simulink model "PV_BAT_GRID_TL"  (R2013a)
settings: Solver=ode23t  StartTime=0.0  StopTime=1  RelTol=1e-3
undefined symbols (not defined in the file): Acid, Lead
libraries: powerlib x39, powerlib_meascontrol x10, simulink x4, electricdrivelib x2, fuzblock x2, powerlib_extras x1
settings Model: Creator=penglei  LastModifiedBy=SRIDHARAN
settings SolverCC: ZeroCrossControl=DisableAll
settings DataIOCC: SignalLoggingSaveFormat=ModelDataLogs
settings OptimizationCC: ExpressionDepthLimit=2147483647
settings DebuggingCC: FcnCallInpInsideContextMsg=UseLocalSettings  StrictBusMsg=Warning
settings GRTTargetCC: CombineOutputUpdateFcns=off  GRTInterface=on

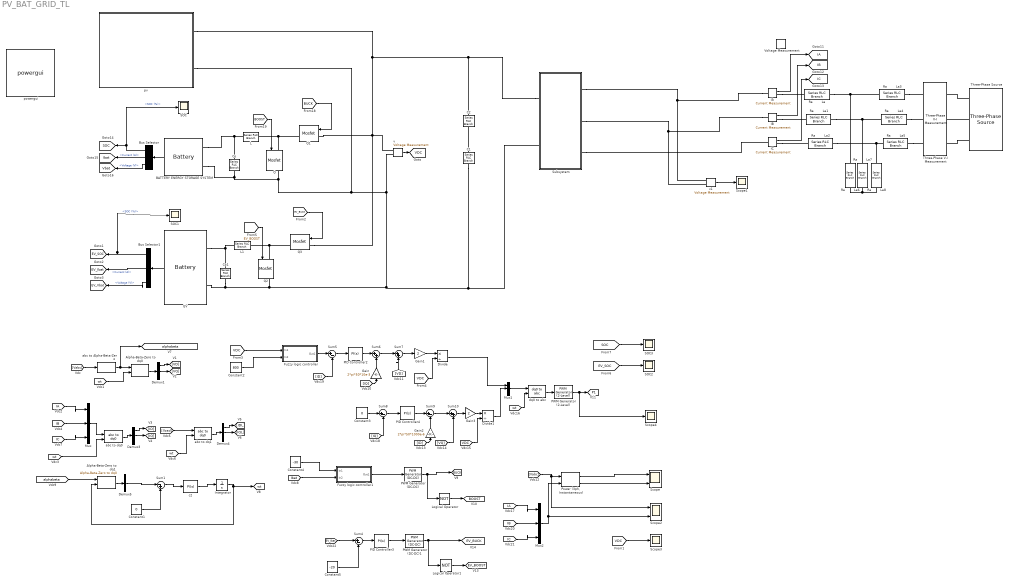
== system PV_BAT_GRID_TL ==
  Alpha-Beta-Zero to dq0 : powerlib_meascontrol/Transformations/Alpha-Beta-Zero to dq0  Alignment=90 degrees behind phase A axis
  Alpha-Beta-Zero to dq1 : powerlib_meascontrol/Transformations/Alpha-Beta-Zero to dq0  Alignment=90 degrees behind phase A axis
  BATTERY ENERGY STORAGE SYSTEM : electricdrivelib/Extra Sources/Battery  BatType=Lead-Acid  ShowDetailedParameters=off  NomV=360  NomQ=300  SOC=50  PresetModel=on  MaxQ=312.5  FullV=391.9737  Dis_rate=60  R=0.012  Normal_OP=93.0833  expZone="[366.5132             1]"  Dis_Char=off  current=[1.5 3]  Units=Ampere-hour  Batt_Tr=1
  Bus Selector : BusSelector  OutputSignals=SOC (%),Current (A),Voltage (V)
  Bus Selector1 : BusSelector  OutputSignals=SOC (%),Current (A),Voltage (V)
  C1 : powerlib/Elements/Series RLC Branch  LConnTagsString=__new0  RConnTagsString=__new0  BranchType=RC  Resistance=1e-3  Inductance=1.0  SetiL0=off  InitialCurrent=0  Capacitance=2500e-6  Setx0=on  InitialVoltage=400  Measurements=None
  C2 : powerlib/Elements/Series RLC Branch  LConnTagsString=__new0  RConnTagsString=__new0  BranchType=RC  Resistance=1e-3  Inductance=1.0  SetiL0=off  InitialCurrent=0  Capacitance=2500e-6  Setx0=on  InitialVoltage=400  Measurements=None
  Co : powerlib/Elements/Series RLC Branch  LConnTagsString=__new0  RConnTagsString=__new0  BranchType=RC  Resistance=0.0001  Inductance=1.0  SetiL0=off  InitialCurrent=0  Capacitance=0.625e-6  Setx0=off  InitialVoltage=0  Measurements=None
  Co1 : powerlib/Elements/Series RLC Branch  LConnTagsString=__new0  RConnTagsString=__new0  BranchType=RC  Resistance=0.0001  Inductance=1.0  SetiL0=off  InitialCurrent=0  Capacitance=0.625e-6  Setx0=off  InitialVoltage=0  Measurements=None
  Constant1 : Constant  Value=0
  Constant2 : Constant  Value=800
  Constant3 : Constant  Value=0
  Constant4 : Constant  Value=-30
  Constant5 : Constant  Value=-20
  Demux{1,3..5} (4 alike) : Demux  Outputs=3
  Divide : Product  Inputs=*/
  Divide1 : Product  Inputs=*/
  EV : electricdrivelib/Extra Sources/Battery  BatType=Lead-Acid  ShowDetailedParameters=off  NomV=48  NomQ=300  SOC=50  PresetModel=on  MaxQ=312.5  FullV=52.2632  Dis_rate=60  R=0.0016  Normal_OP=93.0833  expZone="[48.8684            1]"  Dis_Char=off  current=[1.5 3]  Units=Ampere-hour  Batt_Tr=1
  Fuzzy logic controller : Subsystem
  Fuzzy logic controller1 : Subsystem
  Gain : Gain  Gain=2*pi*50*10e-3
  Gain1 : Gain  Gain=2
  Gain2 : Gain  Gain=2*pi*50*1000e-6
  Gain3 : Gain  Gain=2
  IA : powerlib/Measurements/Current Measurement  PhasorSimulation=off  OutputType=Complex  PSBequivalent=0
  IB : powerlib/Measurements/Current Measurement  PhasorSimulation=off  OutputType=Complex  PSBequivalent=0
  IC : powerlib/Measurements/Current Measurement  PhasorSimulation=off  OutputType=Complex  PSBequivalent=0
  Integrator : Integrator
  L : powerlib/Elements/Series RLC Branch  LConnTagsString=__new0  RConnTagsString=__new0  BranchType=RL  Resistance=0.0001  Inductance=20e-3  SetiL0=off  InitialCurrent=0  Capacitance=1.0  Setx0=off  InitialVoltage=0  Measurements=None
  L1 : powerlib/Elements/Series RLC Branch  LConnTagsString=__new0  RConnTagsString=__new0  BranchType=RL  Resistance=0.0001  Inductance=20e-3  SetiL0=off  InitialCurrent=0  Capacitance=1.0  Setx0=off  InitialVoltage=0  Measurements=None
  Logical Operator : Logic  Operator=NOT  AllPortsSameDT=off  OutDataTypeStr=boolean
  Logical Operator1 : Logic  Operator=NOT  AllPortsSameDT=off  OutDataTypeStr=boolean
  Mux : Mux  Inputs=3
  Mux1 : Mux  Inputs=3
  Mux2 : Mux  Inputs=3
  PID Controller2 : simulink/Continuous/PID Controller  Controller=PI  TimeDomain=Continuous-time  SampleTime=1  IntegratorMethod=Forward Euler  FilterMethod=Forward Euler  Form=Parallel  P=25  I=500  D=0  N=100  InitialConditionSource=internal  InitialConditionForIntegrator=0  InitialConditionForFilter=0  ExternalReset=none  LimitOutput=off  UpperSaturationLimit=1000  LowerSaturationLimit=-1000  LinearizeAsGain=on  AntiWindupMode=none  Kb=1  TrackingMode=off  Kt=1  PParamMin=[]  PParamMax=[]  IParamMin=[]  IParamMax=[]  DParamMin=[]  DParamMax=[]  NParamMin=[]  NParamMax=[]  KbParamMin=[]  KbParamMax=[]  KtParamMin=[]  KtParamMax=[]  POutMin=[]  POutMax=[]  IOutMin=[]  IOutMax=[]  DOutMin=[]  DOutMax=[]  NOutMin=[]  NOutMax=[]  KbOutMin=[]  KbOutMax=[]  KtOutMin=[]  KtOutMax=[]  IntegratorOutMin=[]  IntegratorOutMax=[]  FilterOutMin=[]  FilterOutMax=[]  SumOutMin=[]  SumOutMax=[]  SumI1OutMin=[]  SumI1OutMax=[]  SumI2OutMin=[]  SumI2OutMax=[]  SumI3OutMin=[]  SumI3OutMax=[]  SumDOutMin=[]  SumDOutMax=[]  SaturationOutMin=[]  SaturationOutMax=[]  IntegratorContinuousStateAttributes=''  IntegratorStateMustResolveToSignalObject=off  IntegratorRTWStateStorageClass=Auto  FilterContinuousStateAttributes=''  FilterStateMustResolveToSignalObject=off  FilterRTWStateStorageClass=Auto
  PID Controller3 : simulink/Continuous/PID Controller  Controller=PI  TimeDomain=Continuous-time  SampleTime=1  IntegratorMethod=Forward Euler  FilterMethod=Forward Euler  Form=Parallel  P=0.005  I=10  D=0  N=100  InitialConditionSource=internal  InitialConditionForIntegrator=0  InitialConditionForFilter=0  ExternalReset=none  LimitOutput=on  UpperSaturationLimit=0.95  LowerSaturationLimit=0  LinearizeAsGain=on  AntiWindupMode=none  Kb=1  TrackingMode=off  Kt=1  PParamMin=[]  PParamMax=[]  IParamMin=[]  IParamMax=[]  DParamMin=[]  DParamMax=[]  NParamMin=[]  NParamMax=[]  KbParamMin=[]  KbParamMax=[]  KtParamMin=[]  KtParamMax=[]  POutMin=[]  POutMax=[]  IOutMin=[]  IOutMax=[]  DOutMin=[]  DOutMax=[]  NOutMin=[]  NOutMax=[]  KbOutMin=[]  KbOutMax=[]  KtOutMin=[]  KtOutMax=[]  IntegratorOutMin=[]  IntegratorOutMax=[]  FilterOutMin=[]  FilterOutMax=[]  SumOutMin=[]  SumOutMax=[]  SumI1OutMin=[]  SumI1OutMax=[]  SumI2OutMin=[]  SumI2OutMax=[]  SumI3OutMin=[]  SumI3OutMax=[]  SumDOutMin=[]  SumDOutMax=[]  SaturationOutMin=[]  SaturationOutMax=[]  IntegratorContinuousStateAttributes=''  IntegratorStateMustResolveToSignalObject=off  IntegratorRTWStateStorageClass=Auto  FilterContinuousStateAttributes=''  FilterStateMustResolveToSignalObject=off  FilterRTWStateStorageClass=Auto
  PID Controller4 : simulink/Continuous/PID Controller  Controller=PI  TimeDomain=Continuous-time  SampleTime=1  IntegratorMethod=Forward Euler  FilterMethod=Forward Euler  Form=Parallel  P=25  I=500  D=0  N=100  InitialConditionSource=internal  InitialConditionForIntegrator=0  InitialConditionForFilter=0  ExternalReset=none  LimitOutput=off  UpperSaturationLimit=inf  LowerSaturationLimit=-inf  LinearizeAsGain=on  AntiWindupMode=none  Kb=1  TrackingMode=off  Kt=1  PParamMin=[]  PParamMax=[]  IParamMin=[]  IParamMax=[]  DParamMin=[]  DParamMax=[]  NParamMin=[]  NParamMax=[]  KbParamMin=[]  KbParamMax=[]  KtParamMin=[]  KtParamMax=[]  POutMin=[]  POutMax=[]  IOutMin=[]  IOutMax=[]  DOutMin=[]  DOutMax=[]  NOutMin=[]  NOutMax=[]  KbOutMin=[]  KbOutMax=[]  KtOutMin=[]  KtOutMax=[]  IntegratorOutMin=[]  IntegratorOutMax=[]  FilterOutMin=[]  FilterOutMax=[]  SumOutMin=[]  SumOutMax=[]  SumI1OutMin=[]  SumI1OutMax=[]  SumI2OutMin=[]  SumI2OutMax=[]  SumI3OutMin=[]  SumI3OutMax=[]  SumDOutMin=[]  SumDOutMax=[]  SaturationOutMin=[]  SaturationOutMax=[]  IntegratorContinuousStateAttributes=''  IntegratorStateMustResolveToSignalObject=off  IntegratorRTWStateStorageClass=Auto  FilterContinuousStateAttributes=''  FilterStateMustResolveToSignalObject=off  FilterRTWStateStorageClass=Auto
  PWM Generator (2-Level) : powerlib_meascontrol/Pulse & Signal Generators/PWM Generator (2-Level)  ModulatorType=Three-phase bridge (6 pulses)  ModulatorMode=Unsynchronized  nF=27  Fc=10000  ModulatingSignals=off  m=0.8  Freq=60  Phase=0  Ts=0
  PWM Generator (DC-DC) : powerlib_meascontrol/Pulse & Signal Generators/PWM Generator (DC-DC)  Fsw=10000  Ts=0
  PWM Generator (DC-DC)1 : powerlib_meascontrol/Pulse & Signal Generators/PWM Generator (DC-DC)  Fsw=10000  Ts=0
  "Power (3ph, Instantaneous)" : powerlib_meascontrol/Measurements/Power (3ph, Instantaneous)
  Q{,1..3} (4 alike) : powerlib/Power Electronics/Mosfet  Ron=0.001  Lon=1e-6  Rd=0.001  Vfd=0  IC=0  Rs=1e5  Cs=inf  Measurements=on
  Ra         La{,1..5} (6 alike) : powerlib/Elements/Series RLC Branch  LConnTagsString=__new0  RConnTagsString=__new0  BranchType=L  Resistance=2  Inductance=5e-3  SetiL0=off  InitialCurrent=0  Capacitance=1e-6  Setx0=off  InitialVoltage=0  Measurements=None
  Ra         La6 : powerlib/Elements/Series RLC Branch  LConnTagsString=__new0  RConnTagsString=__new0  BranchType=C  Resistance=2  Inductance=0.01  SetiL0=off  InitialCurrent=0  Capacitance=30e-6  Setx0=off  InitialVoltage=0  Measurements=None
  Ra         La7 : powerlib/Elements/Series RLC Branch  LConnTagsString=__new0  RConnTagsString=__new0  BranchType=C  Resistance=2  Inductance=0.01  SetiL0=off  InitialCurrent=0  Capacitance=30e-6  Setx0=off  InitialVoltage=0  Measurements=None
  Ra         La8 : powerlib/Elements/Series RLC Branch  LConnTagsString=__new0  RConnTagsString=__new0  BranchType=C  Resistance=2  Inductance=0.01  SetiL0=off  InitialCurrent=0  Capacitance=30e-6  Setx0=off  InitialVoltage=0  Measurements=None
  SOC{,1..3} (4 alike) : Scope
      SOC settings: TimeRange=0.1599378881987578  YMin=-40  YMax=40  SaveName=ScopeData5
      SOC1 settings: TimeRange=0.1599378881987578  YMin=-40  YMax=40  SaveName=ScopeData6
      SOC2 settings: TimeRange=0.1599378881987578  YMin=50.0001  YMax=50.0001  SaveName=ScopeData7
      SOC3 settings: TimeRange=0.1599378881987578  YMin=50  YMax=50.0001  SaveName=ScopeData8
  Scope : Scope  NumInputPorts=2
      settings: TimeRange=0.1599378881987578  YMin=-40~-1000  YMax=40~1000
  Scope1 : Scope
      settings: TimeRange=0.1599378881987578  YMin=-900  YMax=900
  Scope2 : Scope  NumInputPorts=2
      settings: TimeRange=0.1739130434782609  YMin=-400~-300  YMax=400~200  SaveName=ScopeData2
  Scope3 : Scope
      settings: TimeRange=0.1599378881987578  YMin=867.1  YMax=868.15  SaveName=ScopeData3
  Scope4 : Scope
      settings: TimeRange=0.1599378881987578  YMin=-40  YMax=40  SaveName=ScopeData4
  Subsystem : Subsystem
  Sum1 : Sum  Inputs=|-+  SampleTime=1e-6
  Sum10 : Sum  Inputs=|++
  Sum{4..5,8..9} (4 alike) : Sum  Inputs=|+-
  Sum6 : Sum  Inputs=|++
  Sum7 : Sum  Inputs=|++
  Three-Phase V-I Measurement : powerlib/Measurements/Three-Phase V-I Measurement  VoltageMeasurement=phase-to-ground  SetLabelV=on  LabelV=Vabc  Vpu=off  VpuLL=off  CurrentMeasurement=no  SetLabelI=off  LabelI=Iabc  Ipu=off  Pbase=100e6  Vbase=500e3  OutputType=Complex  PhasorSimulation=off  PSBequivalent=0
  Three-Phase Source : powerlib/Electrical Sources/Three-Phase Source  Voltage=415  PhaseAngle=0  Frequency=50  InternalConnection=Yg  SpecifyImpedance=off  Resistance=0.8929e-3  Inductance=16.58e-9  ShortCircuitLevel=100e6  BaseVoltage=415  XRratio=7  BusType=swing  Pref=0  Qref=0  Qmin=-inf  Qmax=inf
  Voltage Measurement : powerlib/Measurements/Voltage Measurement  PhasorSimulation=off  OutputType=Complex  PSBequivalent=0
  abc to Alpha-Beta-Zero : powerlib_meascontrol/Transformations/abc to Alpha-Beta-Zero
  abc to dq0 : powerlib_meascontrol/Transformations/abc to dq0  Alignment=90 degrees behind phase A axis
  abc to dq1 : powerlib_meascontrol/Transformations/abc to dq0  Alignment=90 degrees behind phase A axis
  c2 : simulink/Continuous/PID Controller  Controller=PI  TimeDomain=Continuous-time  SampleTime=1e-6  IntegratorMethod=Forward Euler  FilterMethod=Forward Euler  Form=Parallel  P=10  I=50000  D=0  N=100  InitialConditionSource=internal  InitialConditionForIntegrator=0  InitialConditionForFilter=0  ExternalReset=none  LimitOutput=off  UpperSaturationLimit=inf  LowerSaturationLimit=-inf  LinearizeAsGain=on  AntiWindupMode=none  Kb=1  TrackingMode=off  Kt=1  PParamMin=[]  PParamMax=[]  IParamMin=[]  IParamMax=[]  DParamMin=[]  DParamMax=[]  NParamMin=[]  NParamMax=[]  KbParamMin=[]  KbParamMax=[]  KtParamMin=[]  KtParamMax=[]  POutMin=[]  POutMax=[]  IOutMin=[]  IOutMax=[]  DOutMin=[]  DOutMax=[]  NOutMin=[]  NOutMax=[]  KbOutMin=[]  KbOutMax=[]  KtOutMin=[]  KtOutMax=[]  IntegratorOutMin=[]  IntegratorOutMax=[]  FilterOutMin=[]  FilterOutMax=[]  SumOutMin=[]  SumOutMax=[]  SumI1OutMin=[]  SumI1OutMax=[]  SumI2OutMin=[]  SumI2OutMax=[]  SumI3OutMin=[]  SumI3OutMax=[]  SumDOutMin=[]  SumDOutMax=[]  SaturationOutMin=[]  SaturationOutMax=[]  IntegratorContinuousStateAttributes=''  IntegratorStateMustResolveToSignalObject=off  IntegratorRTWStateStorageClass=Auto  FilterContinuousStateAttributes=''  FilterStateMustResolveToSignalObject=off  FilterRTWStateStorageClass=Auto
  dq0 to abc : powerlib_meascontrol/Transformations/dq0 to abc  Alignment=90 degrees behind phase A axis
  powergui : powerlib/powergui  SimulationMode=Discrete  SolverType=Tustin  SampleTime=1e-5  frequency=60  SPID=off  DisableSnubberDevices=off  DisableRonSwitches=off  DisableVfSwitches=off  SwTol=0  Interpol=off  DisplayEquations=off  frequencyindice=0  Pbase=100e6  ErrMax=1e-4  Iterations=50  UnitsV=kV  UnitsW=MW  FunctionMessages=off  echomessages=off  HookPort=off  EnableUseOfTLC=off  x0status=blocks  RestoreLinks=warning  ResistiveCurrentMeasurement=off  Frange=[0:2:500]  Ylog=off  Xlog=on  ShowGrid=off  save=off  variable=ZData  ZoomFFT=on  StartTime=0.0  cycles=1  DisplayStyle=1  fundamental=60  FreqAxis=off  MaxFrequency=1000  frequencyindicesteady=1  RmsSteady=1  display=off  Ts=0  methode=off
  pv : Subsystem
  v : powerlib/Measurements/Voltage Measurement  PhasorSimulation=off  OutputType=Complex  PSBequivalent=0
  v1 : powerlib/Measurements/Voltage Measurement  PhasorSimulation=off  OutputType=Complex  PSBequivalent=0
  tag scope: BOOST=global, BUCK=global, EV_BOOST=global, EV_BUCK=global, EV_Ibat=global, EV_SOC=global, EV_Vbat=global, IA=global, IB=global, IC=global, Ibat=global, P1=global, SOC=global, VDC=global, Vbat=global, alphabeta=global, wt=global
  wires:
  v/1 -> [VDC]
  IA/1 -> [IA]
  IB/1 -> [IB]
  IC/1 -> [IC]
  [BUCK] -> Q1/1
  [BOOST] -> Q/1
  BATTERY ENERGY STORAGE SYSTEM/1 -> Bus Selector/1
  Bus Selector/1 -> SOC/1, [SOC]  "<SOC (%)>"
  Bus Selector/2 -> [Ibat]  "<Current (A)>"
  Bus Selector/3 -> [Vbat]  "<Voltage (V)>"
  [Vabc] -> abc to Alpha-Beta-Zero/1
  abc to Alpha-Beta-Zero/1 -> [alphabeta], Alpha-Beta-Zero to dq0/1
  Alpha-Beta-Zero to dq0/1 -> Demux1/1
  Demux1/2 -> [VQ]
  Demux1/1 -> [VD]
  [wt] -> Alpha-Beta-Zero to dq0/2
  [wt] -> abc to dq0/2
  Demux3/2 -> [IQ]
  Demux3/1 -> [ID]
  abc to dq0/1 -> Demux3/1
  [wt] -> abc to dq1/2
  [Iload] -> abc to dq1/1
  Demux4/2 -> [IQL]
  Demux4/1 -> [IDL]
  abc to dq1/1 -> Demux4/1
  [IB] -> Mux/2
  [IC] -> Mux/3
  [IA] -> Mux/1
  Mux/1 -> abc to dq0/1
  Alpha-Beta-Zero to dq1/1 -> Demux5/1
  Demux5/2 -> Sum1/1
  Integrator/1 -> [wt], Alpha-Beta-Zero to dq1/2
  [alphabeta] -> Alpha-Beta-Zero to dq1/1
  Sum1/1 -> c2/1
  Constant1/1 -> Sum1/2
  c2/1 -> Integrator/1
  [ID] -> Sum5/2
  Sum5/1 -> PID Controller2/1
  PID Controller2/1 -> Sum6/1
  Gain/1 -> Sum6/2
  [IQ] -> Gain/1
  Sum6/1 -> Sum7/1
  [VD] -> Sum7/2
  Sum7/1 -> Gain1/1
  Gain1/1 -> Divide/1
  [VDC] -> Divide/2
  [IQ] -> Sum8/2
  Sum8/1 -> PID Controller4/1
  PID Controller4/1 -> Sum9/1
  Gain2/1 -> Sum9/2
  [ID] -> Gain2/1
  Sum9/1 -> Sum10/1
  [VQ] -> Sum10/2
  Sum10/1 -> Gain3/1
  Gain3/1 -> Divide1/1
  [VDC] -> Divide1/2
  Constant3/1 -> Sum8/1
  Divide/1 -> Mux1/1
  Divide1/1 -> Mux1/2
  Mux1/1 -> dq0 to abc/1
  [wt] -> dq0 to abc/2
  dq0 to abc/1 -> PWM Generator (2-Level)/1
  PWM Generator (DC-DC)/1 -> Logical Operator/1, [BUCK]
  Logical Operator/1 -> [BOOST]
  PWM Generator (2-Level)/1 -> Scope4/1, [P1]
  [Vabc] -> Scope2/1, "Power (3ph, Instantaneous)"/1
  [IB] -> Mux2/2
  [IC] -> Mux2/3
  [IA] -> Mux2/1
  Mux2/1 -> "Power (3ph, Instantaneous)"/2, Scope2/2
  "Power (3ph, Instantaneous)"/2 -> Scope/2
  "Power (3ph, Instantaneous)"/1 -> Scope/1
  [VDC] -> Scope3/1
  v1/1 -> Scope1/1
  [EV_BUCK] -> Q3/1
  [EV_BOOST] -> Q2/1
  EV/1 -> Bus Selector1/1
  Bus Selector1/1 -> [EV_SOC], SOC1/1  "<SOC (%)>"
  Bus Selector1/2 -> [EV_Ibat]  "<Current (A)>"
  Bus Selector1/3 -> [EV_Vbat]  "<Voltage (V)>"
  [EV_Ibat] -> Sum4/1
  Constant5/1 -> Sum4/2
  Sum4/1 -> PID Controller3/1
  PID Controller3/1 -> PWM Generator (DC-DC)1/1
  PWM Generator (DC-DC)1/1 -> [EV_BUCK], Logical Operator1/1
  Logical Operator1/1 -> [EV_BOOST]
  [EV_SOC] -> SOC2/1
  [SOC] -> SOC3/1
  Fuzzy logic controller/1(Out1) -> Sum5/1
  Constant2/1 -> Fuzzy logic controller/2(In2)
  [VDC] -> Fuzzy logic controller/1(In1)
  Fuzzy logic controller1/1(Out1) -> PWM Generator (DC-DC)/1
  [Ibat] -> Fuzzy logic controller1/2(In2)
  Constant4/1 -> Fuzzy logic controller1/1(In1)
  connections:
  Three-Phase Source/RConn2 -- Three-Phase V-I Measurement/RConn2
  Three-Phase Source/RConn3 -- Three-Phase V-I Measurement/RConn3
  Three-Phase Source/RConn1 -- Three-Phase V-I Measurement/RConn1
  BATTERY ENERGY STORAGE SYSTEM/LConn1 -- Co/LConn1 -- L/RConn1
  C1/LConn1 -- C2/RConn1
  Ra         La/RConn1 -- Ra         La6/LConn1 -- Ra         La3/LConn1
  Ra         La3/RConn1 -- Three-Phase V-I Measurement/LConn1
  Ra         La4/RConn1 -- Three-Phase V-I Measurement/LConn2
  Ra         La5/RConn1 -- Three-Phase V-I Measurement/LConn3
  Ra         La1/RConn1 -- Ra         La7/LConn1 -- Ra         La4/LConn1
  Ra         La2/RConn1 -- Ra         La8/LConn1 -- Ra         La5/LConn1
  Ra         La8/RConn1 -- Ra         La6/RConn1 -- Ra         La7/RConn1
  Q/LConn1 -- L/LConn1 -- Q1/RConn1
  IA/RConn1 -- Ra         La/LConn1
  IB/RConn1 -- Ra         La1/LConn1
  IC/RConn1 -- Ra         La2/LConn1
  Subsystem/LConn1 -- Q3/LConn1 -- Q1/LConn1 -- v/LConn1 -- pv/RConn1 -- C2/LConn1
  Co1/RConn1 -- EV/LConn2 -- pv/RConn2 -- Co/RConn1 -- BATTERY ENERGY STORAGE SYSTEM/LConn2 -- Q/RConn1 -- v/LConn2 -- C1/RConn1 -- Subsystem/LConn2 -- Q2/RConn1
  IA/LConn1 -- v1/LConn1 -- Subsystem/RConn1
  IB/LConn1 -- v1/LConn2 -- Subsystem/RConn2
  Subsystem/RConn3 -- IC/LConn1
  EV/LConn1 -- L1/RConn1 -- Co1/LConn1
  Q2/LConn1 -- Q3/RConn1 -- L1/LConn1

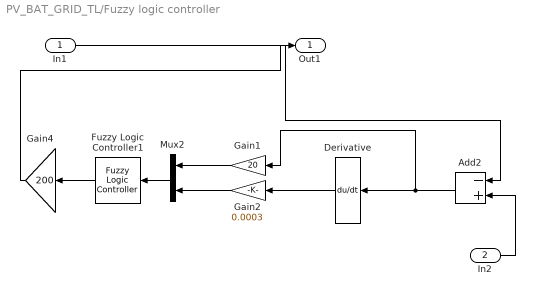
== system PV_BAT_GRID_TL/Fuzzy logic controller ==
  In1 : Inport
  In2 : Inport  Port=2
  Add2 : Sum  Inputs=-+
  Derivative : Derivative
  Fuzzy Logic Controller1 : fuzblock/Fuzzy Logic  Controller  fis=FUZ_BATTERY
  Gain1 : Gain  Gain=20
  Gain2 : Gain  Gain=0.0003
  Gain4 : Gain  Gain=200
  Mux2 : Mux  Inputs=2
  Out1 : Outport
  wires:
  Fuzzy Logic Controller1/1 -> Gain4/1
  Mux2/1 -> Fuzzy Logic Controller1/1
  Gain2/1 -> Mux2/2
  Gain1/1 -> Mux2/1
  Add2/1 -> Derivative/1, Gain1/1
  Derivative/1 -> Gain2/1
  In1/1 -> Add2/1
  Gain4/1 -> Out1/1
  In2/1 -> Add2/2

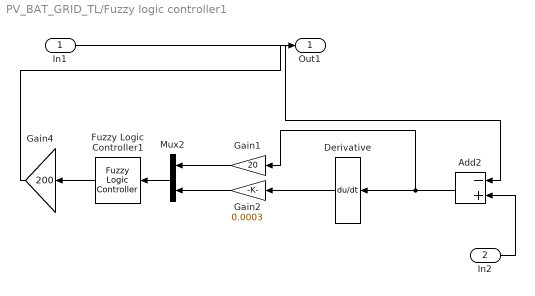
== system PV_BAT_GRID_TL/Fuzzy logic controller1 ==
  In1 : Inport
  In2 : Inport  Port=2
  Add2 : Sum  Inputs=-+
  Derivative : Derivative
  Fuzzy Logic Controller1 : fuzblock/Fuzzy Logic  Controller  fis=FUZ_BATTERY
  Gain1 : Gain  Gain=20
  Gain2 : Gain  Gain=0.0003
  Gain4 : Gain  Gain=200
  Mux2 : Mux  Inputs=2
  Out1 : Outport
  wires:
  In2/1 -> Add2/2
  Gain4/1 -> Out1/1
  In1/1 -> Add2/1
  Derivative/1 -> Gain2/1
  Add2/1 -> Gain1/1, Derivative/1
  Gain1/1 -> Mux2/1
  Gain2/1 -> Mux2/2
  Mux2/1 -> Fuzzy Logic Controller1/1
  Fuzzy Logic Controller1/1 -> Gain4/1

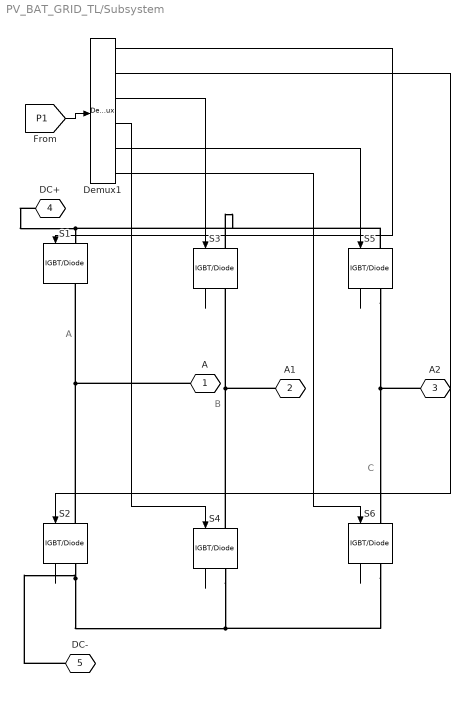
== system PV_BAT_GRID_TL/Subsystem ==
  note: A
  note: B
  note: C
  Demux1 : Demux  Outputs=6
  S{1..6} (6 alike) : powerlib/Power Electronics/IGBT//Diode  Ron=1e-3  Rs=1e5  Cs=inf  Measurements=on
  A : PMIOPort  Tag=PMCPort  Port=1  Side=Right
  A1 : PMIOPort  Tag=PMCPort  Port=2  Side=Right
  A2 : PMIOPort  Tag=PMCPort  Port=3  Side=Right
  DC+ : PMIOPort  Tag=PMCPort  Port=4  Side=Left
  DC- : PMIOPort  Tag=PMCPort  Port=5  Side=Left
  wires:
  Demux1/2 -> S2/1
  Demux1/1 -> S1/1
  [P1] -> Demux1/1
  Demux1/3 -> S3/1
  Demux1/4 -> S4/1
  Demux1/5 -> S5/1
  Demux1/6 -> S6/1
  S3/1 -> ?
  S2/1 -> ?
  S6/1 -> ?
  S5/1 -> ?
  S4/1 -> ?
  connections:
  S2/LConn1 -- A/RConn1 -- S1/RConn1
  S5/RConn1 -- A2/RConn1 -- S6/LConn1
  S4/LConn1 -- A1/RConn1 -- S3/RConn1
  S2/RConn1 -- S6/RConn1 -- S4/RConn1 -- DC-/RConn1
  S5/LConn1 -- S3/LConn1 -- DC+/RConn1 -- S1/LConn1

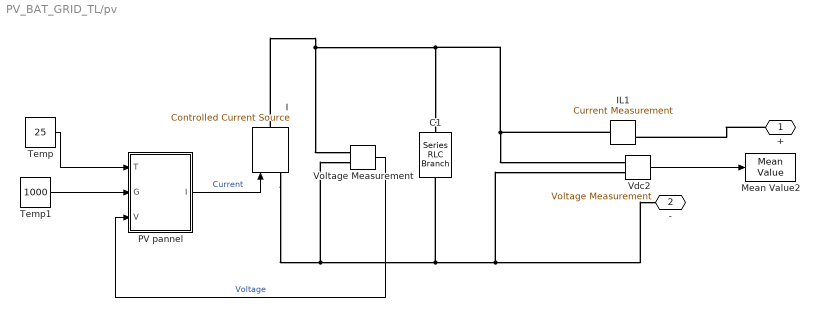
== system PV_BAT_GRID_TL/pv ==
  C1 : powerlib/Elements/Series RLC Branch  LConnTagsString=__new0  RConnTagsString=__new0  BranchType=C  Resistance=0.01  Inductance=1.0  SetiL0=off  InitialCurrent=0  Capacitance=3000e-6  Setx0=off  InitialVoltage=0  Measurements=None
  I : powerlib/Electrical Sources/Controlled Current Source  Initialize=on  Source_Type=AC  Amplitude=0  Phase=0  Frequency=0  Measurements=None
  IL1 : powerlib/Measurements/Current Measurement  PhasorSimulation=off  OutputType=Complex  PSBequivalent=0
  Mean Value2 : powerlib_extras/Measurements/Mean Value  Period=0.0045
  PV pannel : Subsystem  mask(Photovoltaic Pannel :){Ns=50, Voc=64, Isc=5.96, Rs=0.18, Rp=360, se=14, par=30}
      mask prompts: Ns "Number of Series Connected cells"; Voc "Open-circuit voltage"; Isc "Short Circuit Current"; Rs "Series Resistance"; Rp "Parallel Resistance"; se "No: of Modules in Series"; par "No: of Modules in Parallel"
  Temp : Constant  Value=25
  Temp1 : Constant  Value=1000
  Vdc2 : powerlib/Measurements/Voltage Measurement  Tag=PoWeRsYsTeMmEaSuReMeNt  PhasorSimulation=off  OutputType=Magnitude  PSBequivalent=0
  Voltage Measurement : powerlib/Measurements/Voltage Measurement  PhasorSimulation=off  OutputType=Complex  PSBequivalent=0
  + : PMIOPort  Port=1  Side=Right
  - : PMIOPort  Port=2  Side=Right
  wires:
  Vdc2/1 -> Mean Value2/1
  Temp/1 -> PV pannel/1(T)
  Temp1/1 -> PV pannel/2(G)
  PV pannel/1(I) -> I/1  "Current"
  Voltage Measurement/1 -> PV pannel/3(V)  "Voltage"
  connections:
  +/RConn1 -- IL1/RConn1
  IL1/LConn1 -- C1/LConn1 -- I/RConn1 -- Voltage Measurement/LConn1 -- Vdc2/LConn1
  I/LConn1 -- Voltage Measurement/LConn2 -- C1/RConn1 -- -/RConn1 -- Vdc2/LConn2

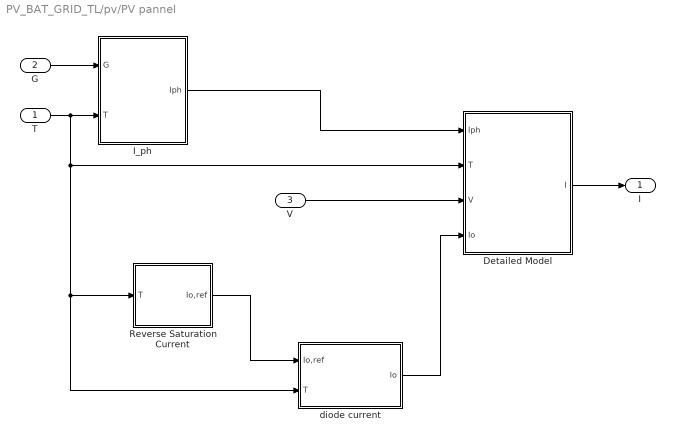
== system PV_BAT_GRID_TL/pv/PV pannel ==
  T : Inport
  G : Inport  Port=2
  V : Inport  Port=3
  Detailed Model : Subsystem
  I_ph : Subsystem
  Reverse Saturation Current : Subsystem
  diode current : Subsystem
  I : Outport
  wires:
  G/1 -> I_ph/1(G)
  T/1 -> I_ph/2(T), Reverse Saturation Current/1(T), diode current/2(T), Detailed Model/2(T)
  diode current/1(Io) -> Detailed Model/4(Io)
  Reverse Saturation Current/1(Io,ref) -> diode current/1(Io,ref)
  V/1 -> Detailed Model/3(V)
  I_ph/1(Iph) -> Detailed Model/1(Iph)
  Detailed Model/1(I) -> I/1

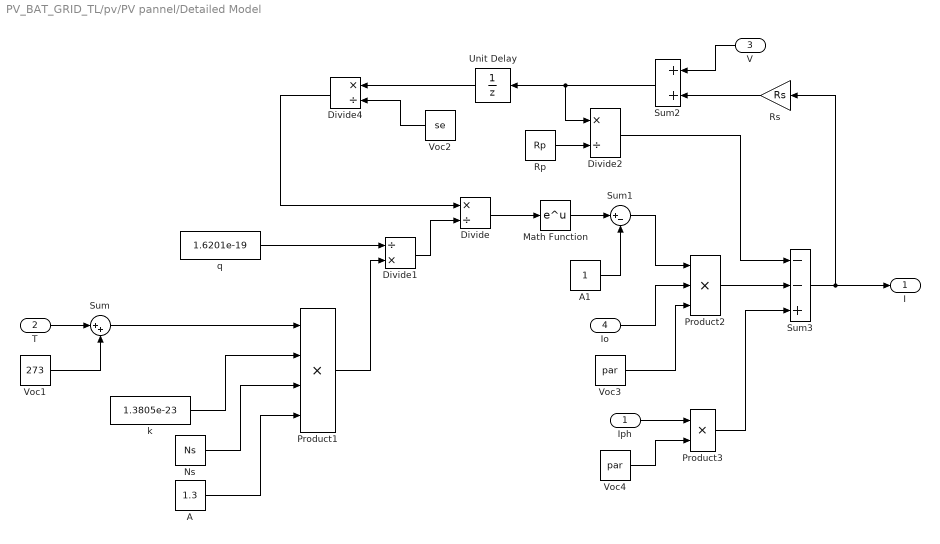
== system PV_BAT_GRID_TL/pv/PV pannel/Detailed Model ==
  Iph : Inport
  T : Inport  Port=2
  V : Inport  Port=3
  Io : Inport  Port=4
  A : Constant  Value=1.3
  A1 : Constant
  Divide : Product  Inputs=*/
  Divide1 : Product  Inputs=/*
  Divide2 : Product  Inputs=*/
  Divide4 : Product  Inputs=*/
  Math Function : Math  SaturateOnIntegerOverflow=on
  Ns : Constant  Value=Ns
  Product1 : Product  Inputs=4  RndMeth=Zero
  Product2 : Product  Inputs=3  RndMeth=Zero
  Product3 : Product  RndMeth=Zero
  Rp : Constant  Value=Rp
  Rs : Gain  Gain=Rs
  Sum : Sum  Inputs=|++
  Sum1 : Sum  Inputs=|+-
  Sum2 : Sum
  Sum3 : Sum  Inputs=--+
  Unit Delay : UnitDelay  SampleTime=-1
  Voc1 : Constant  Value=273
  Voc2 : Constant  Value=se
  Voc3 : Constant  Value=par
  Voc4 : Constant  Value=par
  k : Constant  Value=1.3805e-23
  q : Constant  Value=1.6201e-19
  I : Outport
  wires:
  V/1 -> Sum2/1
  Sum2/1 -> Divide2/1, Unit Delay/1
  Rs/1 -> Sum2/2
  Sum3/1 -> Rs/1, I/1
  Io/1 -> Product2/2
  T/1 -> Sum/1
  Voc1/1 -> Sum/2
  Sum/1 -> Product1/1
  A/1 -> Product1/4
  Ns/1 -> Product1/3
  k/1 -> Product1/2
  Divide/1 -> Math Function/1
  Math Function/1 -> Sum1/1
  A1/1 -> Sum1/2
  Sum1/1 -> Product2/1
  Product2/1 -> Sum3/2
  q/1 -> Divide1/1
  Product1/1 -> Divide1/2
  Divide1/1 -> Divide/2
  Rp/1 -> Divide2/2
  Divide2/1 -> Sum3/1
  Voc3/1 -> Product2/3
  Divide4/1 -> Divide/1
  Voc2/1 -> Divide4/2
  Iph/1 -> Product3/1
  Voc4/1 -> Product3/2
  Product3/1 -> Sum3/3
  Unit Delay/1 -> Divide4/1

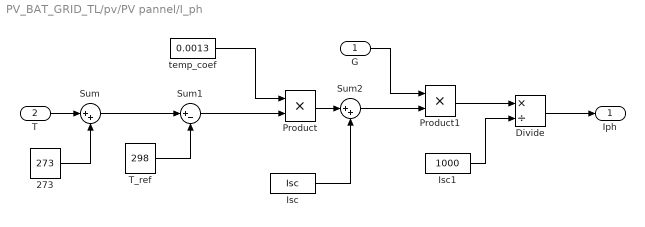
== system PV_BAT_GRID_TL/pv/PV pannel/I_ph ==
  G : Inport
  T : Inport  Port=2
  273 : Constant  Value=273
  Divide : Product  Inputs=*/
  Isc : Constant  Value=Isc
  Isc1 : Constant  Value=1000
  Product : Product  RndMeth=Zero
  Product1 : Product  RndMeth=Zero
  Sum : Sum  Inputs=|++
  Sum1 : Sum  Inputs=|+-
  Sum2 : Sum  Inputs=|++
  T_ref : Constant  Value=298
  temp_coef : Constant  Value=0.0013
  Iph : Outport
  wires:
  T/1 -> Sum/1
  273/1 -> Sum/2
  Sum/1 -> Sum1/1
  T_ref/1 -> Sum1/2
  Sum1/1 -> Product/2
  temp_coef/1 -> Product/1
  Product/1 -> Sum2/1
  Isc/1 -> Sum2/2
  Sum2/1 -> Product1/2
  G/1 -> Product1/1
  Product1/1 -> Divide/1
  Isc1/1 -> Divide/2
  Divide/1 -> Iph/1

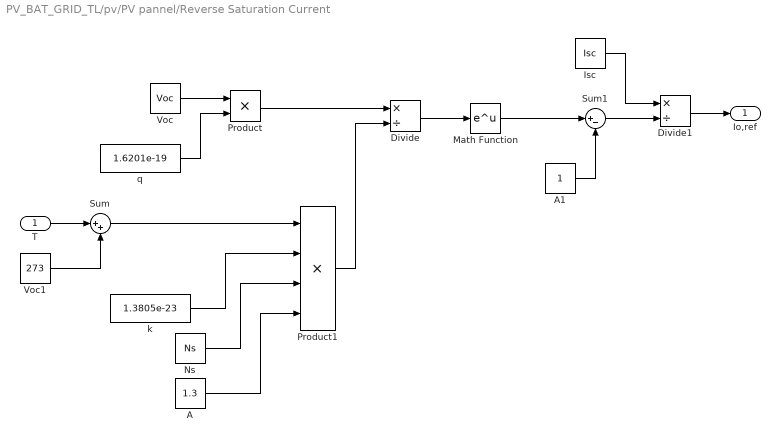
== system PV_BAT_GRID_TL/pv/PV pannel/Reverse Saturation Current ==
  T : Inport
  A : Constant  Value=1.3
  A1 : Constant
  Divide : Product  Inputs=*/
  Divide1 : Product  Inputs=*/
  Isc : Constant  Value=Isc
  Math Function : Math  SaturateOnIntegerOverflow=on
  Ns : Constant  Value=Ns
  Product : Product  RndMeth=Zero
  Product1 : Product  Inputs=4  RndMeth=Zero
  Sum : Sum  Inputs=|++
  Sum1 : Sum  Inputs=|+-
  Voc : Constant  Value=Voc
  Voc1 : Constant  Value=273
  k : Constant  Value=1.3805e-23
  q : Constant  Value=1.6201e-19
  Io,ref : Outport
  wires:
  Voc/1 -> Product/1
  q/1 -> Product/2
  Product/1 -> Divide/1
  T/1 -> Sum/1
  Voc1/1 -> Sum/2
  Sum/1 -> Product1/1
  A/1 -> Product1/4
  Ns/1 -> Product1/3
  k/1 -> Product1/2
  Product1/1 -> Divide/2
  Divide/1 -> Math Function/1
  Math Function/1 -> Sum1/1
  A1/1 -> Sum1/2
  Sum1/1 -> Divide1/2
  Isc/1 -> Divide1/1
  Divide1/1 -> Io,ref/1

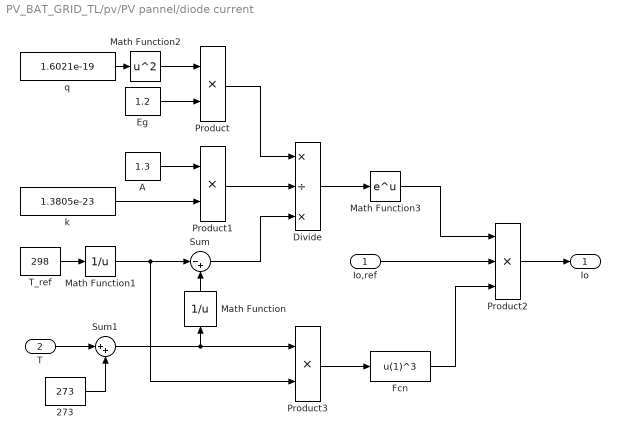
== system PV_BAT_GRID_TL/pv/PV pannel/diode current ==
  Io,ref : Inport
  T : Inport  Port=2
  273 : Constant  Value=273
  A : Constant  Value=1.3
  Divide : Product  Inputs=*/*
  Eg : Constant  Value=1.2
  Fcn : Fcn  Expr=u(1)^3
  Math Function : Math  Operator=reciprocal  SaturateOnIntegerOverflow=on
  Math Function1 : Math  Operator=reciprocal  SaturateOnIntegerOverflow=on
  Math Function2 : Math  Operator=square  SaturateOnIntegerOverflow=on
  Math Function3 : Math  SaturateOnIntegerOverflow=on
  Product : Product  RndMeth=Zero
  Product1 : Product  RndMeth=Zero
  Product2 : Product  Inputs=3  RndMeth=Zero
  Product3 : Product  RndMeth=Zero
  Sum : Sum  Inputs=|-+
  Sum1 : Sum  Inputs=|++
  T_ref : Constant  Value=298
  k : Constant  Value=1.3805e-23
  q : Constant  Value=1.6021e-19
  Io : Outport
  wires:
  T_ref/1 -> Math Function1/1
  Math Function/1 -> Sum/2
  Math Function1/1 -> Sum/1, Product3/2
  q/1 -> Math Function2/1
  Eg/1 -> Product/2
  A/1 -> Product1/1
  k/1 -> Product1/2
  Product/1 -> Divide/1
  Product1/1 -> Divide/2
  Sum/1 -> Divide/3
  Math Function2/1 -> Product/1
  Divide/1 -> Math Function3/1
  T/1 -> Sum1/1
  Sum1/1 -> Math Function/1, Product3/1
  273/1 -> Sum1/2
  Product3/1 -> Fcn/1
  Fcn/1 -> Product2/3
  Math Function3/1 -> Product2/1
  Io,ref/1 -> Product2/2
  Product2/1 -> Io/1
